simulink model "superstate_example"  (R2016a)
settings: Solver=FixedStepAuto  StartTime=0.0  StopTime=2  FixedStep=0.01  RelTol=1e-3
settings Model: Creator=eispin  LastModifiedBy=eispin

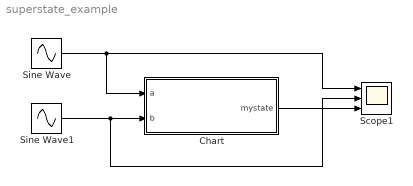
== system superstate_example ==
  Chart : Stateflow chart  TreatAsAtomicUnit=on
  Scope1 : Scope  NumInputPorts=3
  Sine Wave : Sin  Frequency=(3/4)*2*pi  SampleTime=0
  Sine Wave1 : Sin  Frequency=pi  SampleTime=0
  wires:
  Sine Wave/1 -> Scope1/1, Chart/1(a)
  Sine Wave1/1 -> Scope1/2, Chart/2(b)
  Chart/1(mystate) -> Scope1/3

== stateflow chart superstate_example/Chart ==
  state Normal
    state BPos
      en:
      mystate = 3
    state BNeg
      en:
      mystate = 2
    (default) -> BNeg
    BNeg -> BPos : [b > 0]
    BPos -> BNeg : [b < 0]
  state ANegPeak
    en:
    mystate = 1
  (default) -> ANegPeak
  ANegPeak -> Normal : [a > -0.8]
  Normal -> ANegPeak : [a < -0.8]
  data: a input; b input; mystate output
